simulink model "bikeModel"  (R2024a)
settings: Solver=VariableStepAuto  StartTime=0.0  StopTime=10.0  RelTol=1e-3
settings Model: Creator=rodri  LastModifiedBy=rodri

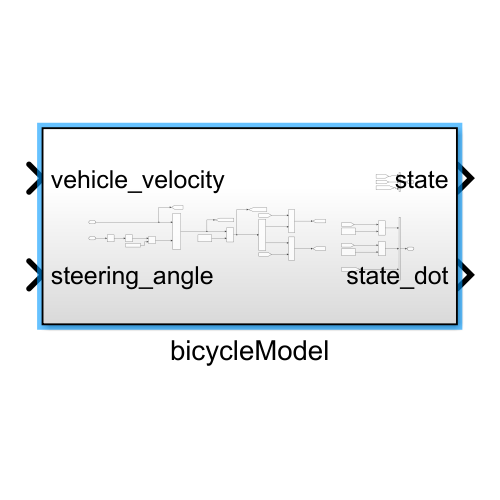
[thumbnail: Simulink's stored preview of the top-level diagram]
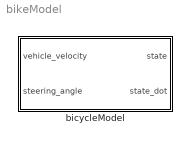
== system bikeModel ==
  bicycleModel : Subsystem

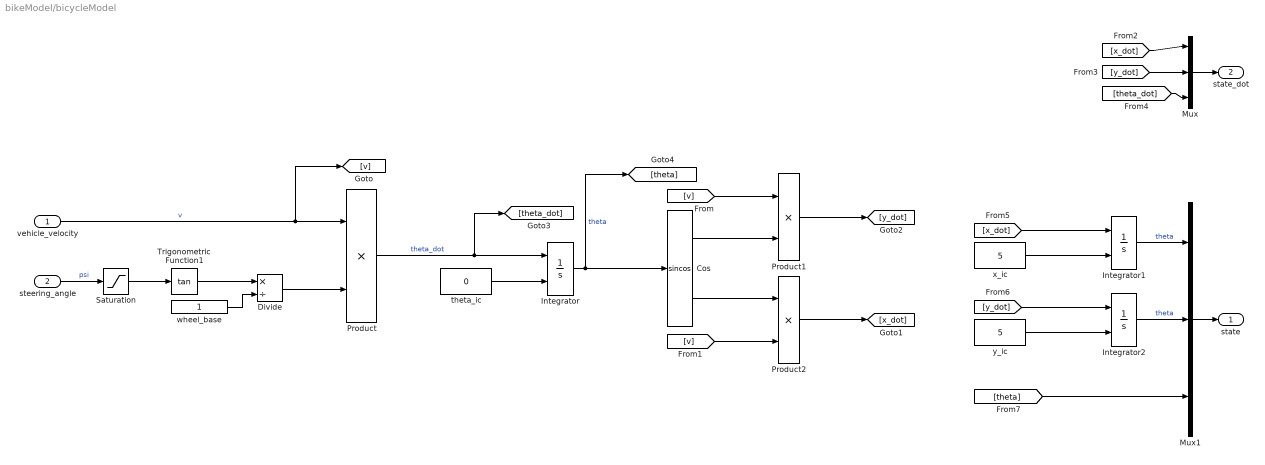
== system bikeModel/bicycleModel ==
  vehicle_velocity : Inport
  steering_angle : Inport  Port=2
  Cos : Trigonometry  Operator=sincos  ApproximationMethod=Lookup  NumberOfDataPoints=32
  Divide : Product  Inputs=*/
  Integrator : Integrator  InitialConditionSource=external
  Integrator1 : Integrator  InitialConditionSource=external
  Integrator2 : Integrator  InitialConditionSource=external
  Mux : Mux  Inputs=3
  Mux1 : Mux  Inputs=3
  Product : Product
  Product1 : Product
  Product2 : Product
  Saturation : Saturate  UpperLimit=pi/3  LowerLimit=0
  Trigonometric Function1 : Trigonometry  Operator=tan
  theta_ic : Constant  Value=0
  wheel_base : Constant
  x_ic : Constant  Value=5
  y_ic : Constant  Value=5
  state : Outport
  state_dot : Outport  Port=2
  wires:
  steering_angle/1 -> Saturation/1  "psi"
  Trigonometric Function1/1 -> Divide/1
  vehicle_velocity/1 -> [v], Product/1  "v"
  Divide/1 -> Product/2
  Product/1 -> [theta_dot], Integrator/1  "theta_dot"
  Integrator/1 -> [theta], Cos/1  "theta"
  theta_ic/1 -> Integrator/2
  Cos/1 -> Product1/2
  Cos/2 -> Product2/1
  [v] -> Product1/1
  [v] -> Product2/2
  Product1/1 -> [y_dot]
  Product2/1 -> [x_dot]
  Mux/1 -> state_dot/1
  [x_dot] -> Mux/1
  [y_dot] -> Mux/2
  [theta_dot] -> Mux/3
  Mux1/1 -> state/1
  [theta] -> Mux1/3
  Integrator1/1 -> Mux1/1  "theta"
  Integrator2/1 -> Mux1/2  "theta"
  [x_dot] -> Integrator1/1
  [y_dot] -> Integrator2/1
  y_ic/1 -> Integrator2/2
  x_ic/1 -> Integrator1/2
  wheel_base/1 -> Divide/2
  Saturation/1 -> Trigonometric Function1/1
